simulink model "MMS_ESC_B_dither_free"  (R2019b)
settings: Solver=ode4  StartTime=par.sym.TStart  StopTime=par.sym.TStop  FixedStep=par.sym.max_dt  MaxStep=par.sym.max_dt  RelTol=1e-3
undefined symbols (not defined in the file): a1_B, amp_B, b, B_0, B_init, K, k, k_B, m, N_buff, N_delay, omega_B, par, R_B, Sat, T_tran, w_L, w_wav
libraries: simulink x1
settings Model: Creator=Vitù  LastModifiedBy=User
settings DataIOCC: SaveFormat=Array  SaveOutput=off  SignalLogging=off  DSMLogging=off  ReturnWorkspaceOutputs=off  TimeSaveName=TIME  OutputSaveName=Yout  OutputOption=SpecifiedOutputTimes  OutputTimes=[par.sym.TStart:par.sym.Outputdt:par.sym.TStop]
settings OptimizationCC: ExpressionDepthLimit=2147483647  LifeSpan=inf
settings DebuggingCC: UnderspecifiedInitializationDetection=Classic  MergeDetectMultiDrivingBlocksExec=none  SolverPrmCheckMsg=warning  AllowSymbolicDim=off  StateNameClashWarn=warning  SFUnexpectedBacktrackingDiag=warning  SFNoUnconditionalDefaultTransitionDiag=warning  SFExecutionAtInitializationDiag=none  ArithmeticOperatorsInVariantConditions=warning
settings HardwareCC: ProdBitPerPointer=32  ProdBitPerSizeT=32  ProdBitPerPtrDiffT=32  ProdLargestAtomicFloat=None  ProdIntDivRoundTo=Undefined  ProdEndianess=Unspecified  ProdWordSize=32  ProdHWDeviceType=32-bit Generic
settings ModelReferenceCC: PropagateSignalLabelsOutOfModel=off
settings SFSimCC: SimUseLocalCustomCode=off  CustomCodeUndefinedFunction=UseInterfaceOnly
settings RTWCC: RTWUseLocalCustomCode=off
settings CodeAppCC: StateflowObjectComments=on
settings GRTTargetCC: TargetLangStandard=C89/C90 (ANSI)  GeneratePreprocessorConditionals=Disable all
settings ConfigComp: CovMetricSettings=dw  CovHtmlReporting=on  CovSaveCumulativeToWorkspaceVar=on  CovSaveSingleToWorkspaceVar=on  CovExternalEMLEnable=off  CovSFcnEnable=off
settings SimscapeCC: SimscapeNormalizeSystem=off
settings ConfigurationSet: Description=SimMechanics 2G

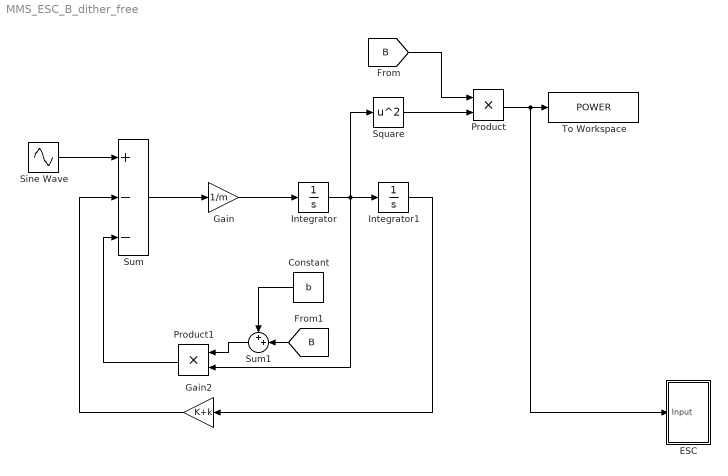
== system MMS_ESC_B_dither_free ==
  Constant : Constant  Value=b
  ESC : Subsystem
  Gain : Gain  Gain=1/m
  Gain2 : Gain  Gain=K+k
  Integrator : Integrator
  Integrator1 : Integrator
  Product : Product
  Product1 : Product
  Sine Wave : Sin  Amplitude=par.H  Frequency=w_wav  SampleTime=0
  Square : Math  Operator=square  SignedPower=off  SaturateOnIntegerOverflow=on
  Sum : Sum  Inputs=+--
  Sum1 : Sum  Inputs=++|
  To Workspace : ToWorkspace  VariableName=POWER  SampleTime=-1
  wires:
  Integrator1/1 -> Gain2/1
  Product/1 -> ESC/1(Input), To Workspace/1
  Product1/1 -> Sum/3
  Gain/1 -> Integrator/1
  Square/1 -> Product/2
  Sum/1 -> Gain/1
  Integrator/1 -> Product1/2, Square/1, Integrator1/1
  Gain2/1 -> Sum/2
  Sine Wave/1 -> Sum/1
  [B] -> Product/1
  [B] -> Sum1/2
  Sum1/1 -> Product1/1
  Constant/1 -> Sum1/1

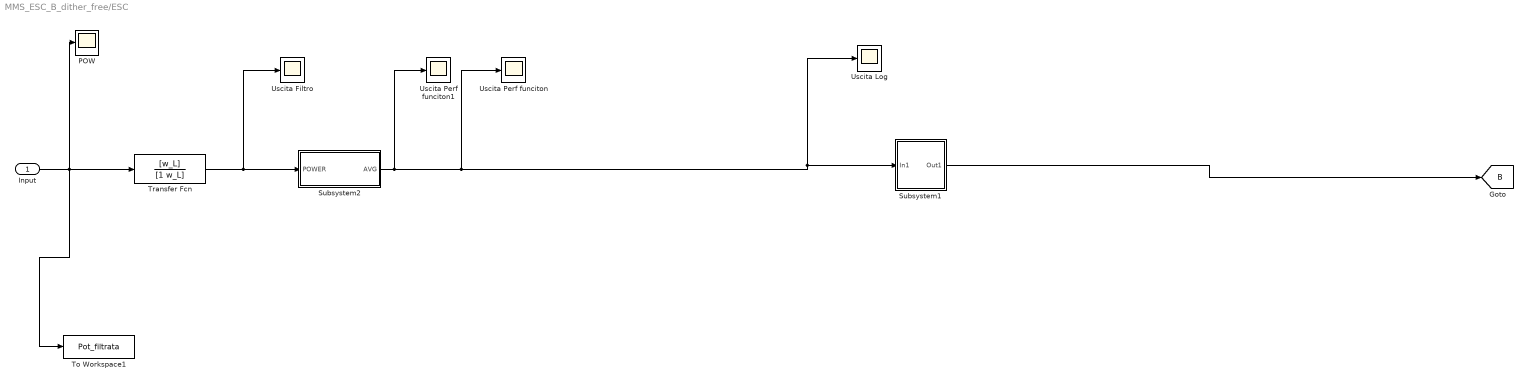
== system MMS_ESC_B_dither_free/ESC ==
  Input : Inport
  POW : Scope
  Subsystem1 : Subsystem
  Subsystem2 : Subsystem
  To Workspace1 : ToWorkspace  VariableName=Pot_filtrata  SampleTime=-1
  Transfer Fcn : TransferFcn  Numerator=[w_L]  Denominator=[1 w_L]
  Uscita Filtro : Scope
  Uscita Log : Scope
  Uscita Perf funciton : Scope
  Uscita Perf funciton1 : Scope
  tag scope: B=global
  wires:
  Input/1 -> POW/1, Transfer Fcn/1, To Workspace1/1
  Subsystem1/1(Out1) -> [B]
  Subsystem2/1(AVG) -> Uscita Perf funciton/1, Uscita Log/1, Subsystem1/1(In1), Uscita Perf funciton1/1
  Transfer Fcn/1 -> Uscita Filtro/1, Subsystem2/1(POWER)

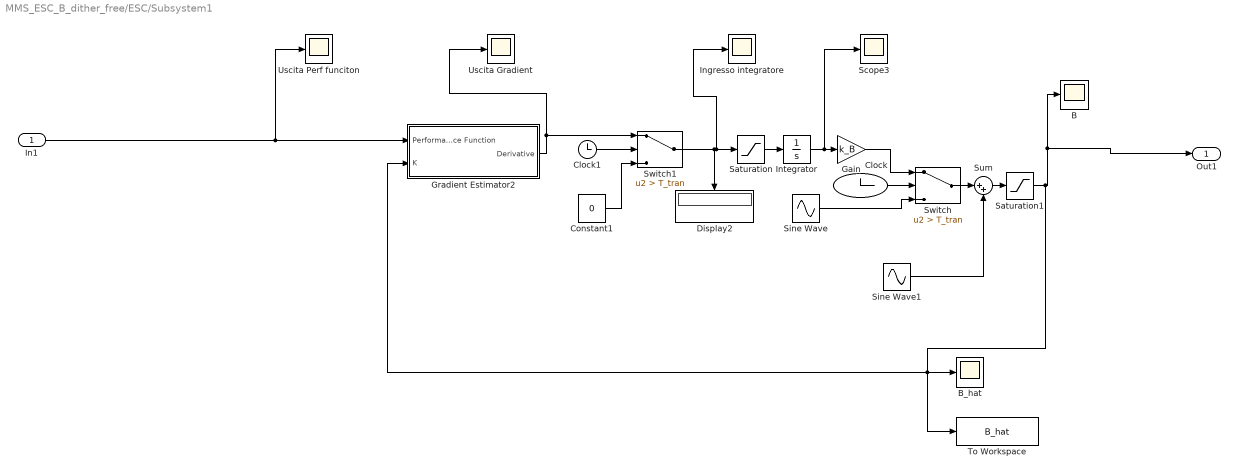
== system MMS_ESC_B_dither_free/ESC/Subsystem1 ==
  In1 : Inport
  B : Scope
  B_hat : Scope
  Clock : Clock
  Clock1 : Clock
  Constant1 : Constant  Value=0
  Display2 : Display
  Gain : Gain  Gain=k_B
  Gradient Estimator2 : Subsystem
  Ingresso integratore : Scope
  Integrator : Integrator  InitialCondition=B_init
  Saturation : Saturate  UpperLimit=Sat  LowerLimit=-Sat
  Saturation1 : Saturate  UpperLimit=inf  LowerLimit=-b
  Scope3 : Scope
  Sine Wave : Sin  Amplitude=a1_B  Bias=B_0  Frequency=w_wav  SampleTime=0
  Sine Wave1 : Sin  Amplitude=amp_B  Frequency=omega_B  SampleTime=0
  Sum : Sum  Inputs=|++
  Switch : Switch  Criteria=u2 > Threshold  Threshold=T_tran
  Switch1 : Switch  Criteria=u2 > Threshold  Threshold=T_tran
  To Workspace : ToWorkspace  VariableName=B_hat  SampleTime=-1
  Uscita Gradient : Scope
  Uscita Perf funciton : Scope
  Out1 : Outport
  wires:
  Sum/1 -> Saturation1/1
  Integrator/1 -> Scope3/1, Gain/1
  Switch/1 -> Sum/1
  Gradient Estimator2/1(Derivative) -> Uscita Gradient/1, Switch1/1
  Clock/1 -> Switch/2
  Sine Wave1/1 -> Sum/2
  In1/1 -> Uscita Perf funciton/1, Gradient Estimator2/1(Performance Function)
  Constant1/1 -> Switch1/3
  Sine Wave/1 -> Switch/3
  Gain/1 -> Switch/1
  Switch1/1 -> Saturation/1, Ingresso integratore/1, Display2/1
  Clock1/1 -> Switch1/2
  Saturation/1 -> Integrator/1
  Saturation1/1 -> Out1/1, B/1, Gradient Estimator2/2(K), To Workspace/1, B_hat/1

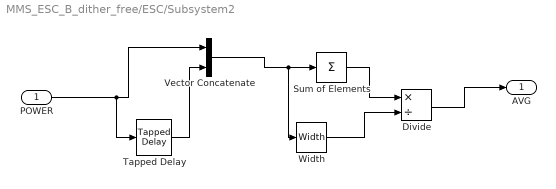
== system MMS_ESC_B_dither_free/ESC/Subsystem2 ==
  POWER : Inport
  Divide : Product  Inputs=*/
  Sum of Elements : Sum  Inputs=+
  Tapped Delay : simulink/Discrete/Tapped Delay  vinit=0  samptime=-1  NumDelays=N_delay  DelayOrder=Oldest  includeCurrent=off
  Vector Concatenate : Concatenate
  Width : Width
  AVG : Outport
  wires:
  POWER/1 -> Tapped Delay/1, Vector Concatenate/1
  Tapped Delay/1 -> Vector Concatenate/2
  Vector Concatenate/1 -> Width/1, Sum of Elements/1
  Sum of Elements/1 -> Divide/1
  Width/1 -> Divide/2
  Divide/1 -> AVG/1

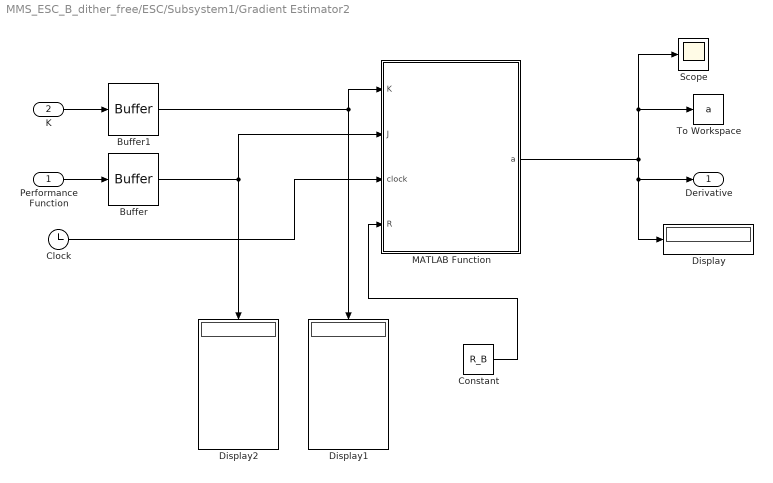
== system MMS_ESC_B_dither_free/ESC/Subsystem1/Gradient Estimator2 ==
  Performance Function : Inport  SampleTime=1
  K : Inport  Port=2  SampleTime=1
  Buffer : Buffer  N=N_buff  V=N_buff-1  OutputFrames=off
  Buffer1 : Buffer  N=N_buff  V=N_buff-1  OutputFrames=off
  Clock : Clock
  Constant : Constant  Value=R_B
  Display : Display
  Display1 : Display
  Display2 : Display
  MATLAB Function : MATLAB Function  TreatAsAtomicUnit=on
  Scope : Scope
  To Workspace : ToWorkspace  VariableName=a  SaveFormat=Timeseries  SampleTime=-1
  Derivative : Outport
  wires:
  MATLAB Function/1(a) -> To Workspace/1, Scope/1, Display/1, Derivative/1
  Performance Function/1 -> Buffer/1
  K/1 -> Buffer1/1
  Buffer/1 -> MATLAB Function/2(J), Display2/1
  Clock/1 -> MATLAB Function/3(clock)
  Buffer1/1 -> Display1/1, MATLAB Function/1(K)
  Constant/1 -> MATLAB Function/4(R)

== matlab function MMS_ESC_B_dither_free/ESC/Subsystem1/Gradient Estimator2/MATLAB Function ==
  data: K input; J input; clock input; a output; R input

function a = LSQ(K,J,clock,R)
if clock > 5
    p = polyfit(K,J,1);
    v = p(1);
%    l = max( [-(log(abs(v))) 9]);
%    l = -log(abs(v));
%     if l<0
%         l=0;
%     end
%   v = v*10^(l);
    s = sign(v);
%    v=abs(v);
%    v = min([v 0.5]);
    a = R*s;
else
    a = 0;
    %l=0;
end

end
